simulink model "pressureSwitch"  (R2014b)
settings: Solver=ode3  SolverMode=SingleTasking  StartTime=0.0  StopTime=inf  RelTol=1e-3
libraries: arduinolib x2
settings Model: ExtModeTrigDuration=2  Creator=The MathWorks Inc.  LastModifiedBy=zpeters
settings DataIOCC: SignalLoggingSaveFormat=ModelDataLogs
settings OptimizationCC: ExpressionDepthLimit=2147483647  OptimizeModelRefInitCode=on  LifeSpan=1
settings DebuggingCC: UnderspecifiedInitializationDetection=Classic  MergeDetectMultiDrivingBlocksExec=none  SolverPrmCheckMsg=none  InheritedTsInSrcMsg=none  ParameterPrecisionLossMsg=none  FcnCallInpInsideContextMsg=EnableAllAsWarning  StateNameClashWarn=warning
settings HardwareCC: ProdBitPerInt=16  ProdBitPerPointer=8  ProdIntDivRoundTo=Zero  ProdEndianess=LittleEndian  ProdWordSize=8  ProdHWDeviceType=Atmel->AVR
settings RTWCC: SystemTargetFile=realtime.tlc  GenerateMakefile=off  TemplateMakefile=realtime.tmf  Description=Run on Target Hardware  RTWVerbose=off  ProcessScript=realtime_make_rtw_hook
settings CodeAppCC: CustomSymbolStrType=$N$R$M  InternalIdentifier=Classic
settings STFCustomTargetCC: TargetLibSuffix=.a  GenerateSampleERTMain=on  ERTCustomFileBanners=on  SupportNonInlinedSFcns=off  SupportVariableSizeSignals=on  MATLABClassNameForMDSCustomization=Simulink.SoftwareTarget.ERTCustomization  GRTInterface=off  SystemTargetFile=realtime.tlc
settings ERTTargetCC: GenerateSampleERTMain=on  ParMdlRefBuildCompliant=off  CompOptLevelCompliant=off  ConcurrentExecutionCompliant=off  CombineOutputUpdateFcns=off  ERTFirstTimeCompliant=off  SupportContinuousTime=on  SupportVariableSizeSignals=on  ModelStepFunctionPrototypeControlCompliant=off  CPPClassGenCompliant=off  ExtModeTransport=3  ExtModeMexFile=ext_serial_win32_comm  ExtModeMexArgs=0 1 9600  InlinedParameterPlacement=NonHierarchical  ERTSrcFileBannerTemplate=realtime_code_template.cgt  ERTHdrFileBannerTemplate=realtime_code_template.cgt  ERTDataSrcFileTemplate=realtime_code_template.cgt  ERTDataHdrFileTemplate=realtime_code_template.cgt  ERTCustomFileTemplate=realtime_file_process.tlc

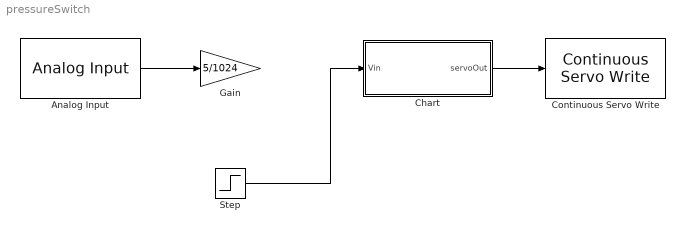
== system pressureSwitch ==
  Analog Input : arduinolib/Analog Input  pinNumber=4  sampleTime=1  blockPlatform=arduino
  Chart : Stateflow chart  TreatAsAtomicUnit=on
  Continuous Servo Write : arduinolib/Continuous Servo Write  pinNumber=4  blockPlatform=arduino
  Gain : Gain  Gain=5/1024
  Step : Step  Time=5  After=5  SampleTime=0
  wires:
  Step/1 -> Chart/1(Vin)
  Chart/1(servoOut) -> Continuous Servo Write/1
  Analog Input/1 -> Gain/1

== stateflow chart pressureSwitch/Chart ==
  state noOp
    en: servoOut = uint8(0);
  state raiseFlag
    en: servoOut = uint8(10);
  state stop
    en: servoOut = uint8(0);
  (default) -> noOp
  noOp -> raiseFlag : [Vin > 2]
  raiseFlag -> stop : [after(10,sec)]
  data: Vin input; servoOut output uint8
